simulink model "PI_current_IM"  (R2018b)
settings: Solver=ode45  StartTime=0.0  StopTime=2  RelTol=1e-7
values from neighbouring files (symbols this model uses):
  fs = 10000    [Motor_parameters_project.m]
  In = 189    [Motor_parameters_project.m]
  J = 0.0151    [Motor_parameters_project.m]
  Ki_d = 15.708    [Motor_parameters_project.m]
  Ki_q = 15.708    [Motor_parameters_project.m]
  Ki_speed = 2    [Motor_parameters_project.m]
  Kp_d = 2.5834    [Motor_parameters_project.m]
  Kp_q = 2.5834    [Motor_parameters_project.m]
  Kp_speed = 2    [Motor_parameters_project.m]
  landa_r = 0.0567    [Motor_parameters_project.m]
  Lm = 0.38e-3    (= 0.00038)    [Motor_parameters_project.m]
  Lr = Lm + Ldr    (= 0.00041116)    [Motor_parameters_project.m]
  Ls = Lm + Lds    (= 0.00041116)    [Motor_parameters_project.m]
  Omegae = 2*pi*fn    (= 364.424747816)    [Motor_parameters_project.m]
  p = 2.0    (= 2)    [Motor_parameters_project.m]
  Rr = 2.69e-3    (= 0.00269)    [Motor_parameters_project.m]
  Rs = 2.5e-3    (= 0.0025)    [Motor_parameters_project.m]
  T_rated = Pn/(2*pi*nn/60)    (= 30.0363631473)    [Motor_parameters_project.m]
  Ts = 1/fs    (= 0.0001)    [Motor_parameters_project.m]
  Udc = 36    [Motor_parameters_project.m]
  Un = 24/sqrt(3)    [Motor_parameters_project.m]
undefined symbols (not defined in the file or in its folder): sigbuilder_block
libraries: powerlib_meascontrol x1, powerlib x1
settings Model: Creator=estef  LastModifiedBy=estef

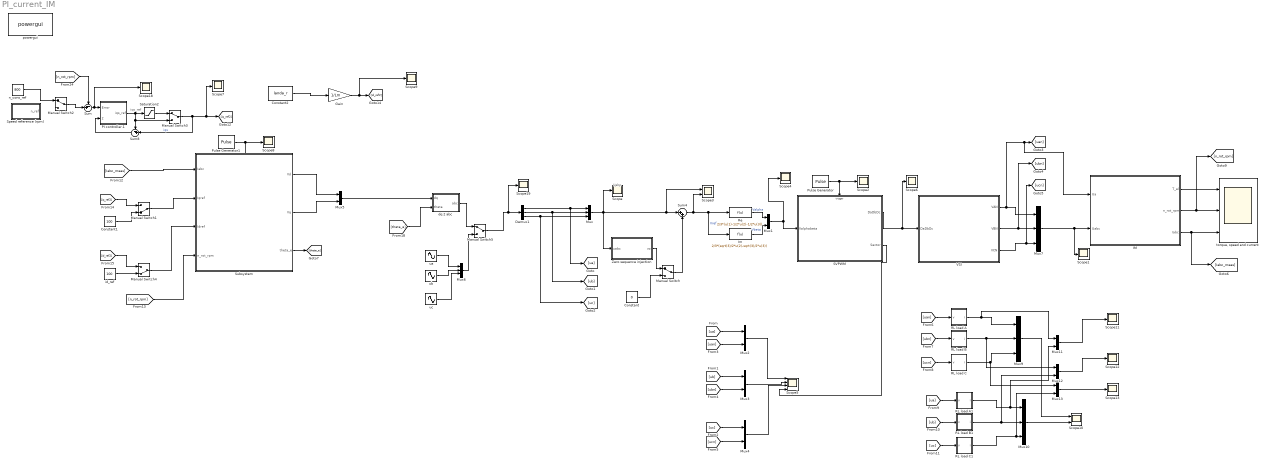
== system PI_current_IM ==
  note: Uabc
  note: iqs_ref
  Constant : Constant  Value=0
  Constant1 : Constant  Value=100
  Constant2 : Constant  Value=landa_r
  Demux1 : Demux  Outputs=3
  Gain : Gain  Gain=1/Lm
  "IM " : Subsystem
  Im : Fcn  Expr=2/3*(sqrt(3)/2*u(2)-sqrt(3)/2*u(3))
  Manual Switch{,2..3,5} (4 alike) : ManualSwitch
  Manual Switch1 : ManualSwitch  CurrentSetting=0
  Manual Switch4 : ManualSwitch  CurrentSetting=0
  Mux{,6..7,9..10} (5 alike) : Mux  Inputs=3
  Mux{1..5,11..13} (8 alike) : Mux  Inputs=2
  PI controller.1 : Subsystem
  Pulse Generator : DiscretePulseGenerator  PulseType=Time based  Period=1/fs  PulseWidth=50  PhaseDelay=1/fs/4
  Pulse Generator1 : DiscretePulseGenerator  PulseType=Time based  Period=2*Ts  PulseWidth=50  PhaseDelay=1/fs/4
  RL load A : Subsystem
  RL load A1 : Subsystem
  RL load B : Subsystem
  RL load B1 : Subsystem
  RL load C : Subsystem
  RL load C1 : Subsystem
  Re : Fcn  Expr=2/3*(u(1)-1/2*u(2)-1/2*u(3))
  "SVPWM " : Subsystem
  Saturation2 : Saturate  UpperLimit=In*sqrt(2)  LowerLimit=-In*sqrt(2)
  Scope{,1..2,4,6..9,11..13,18..19} (13 alike) : Scope
  Scope10 : Scope  NumInputPorts=2
  Scope3 : Scope  NumInputPorts=2
  Scope5 : Scope  NumInputPorts=4
  Speed reference (rpm) : Subsystem  Tag=STV Subsys  LoadFcn=sigbuilder_block('load');  StartFcn=sigbuilder_block('start');  StopFcn=sigbuilder_block('stop');  ClipboardFcn=sigbuilder_block('clipboard');  mask(Sigbuilder block){tuvar=[0:10]}
      mask help: Sigbuilder GUI
      mask init:
      | if ~strcmp(get_param(bdroot(gcbh),'SimulationStatus'),'stopped') tuvar = sigbuilder_block('maskInit'); end
      settings: CopyFcn=sigbuilder_block('copy');  DeleteFcn=sigbuilder_block('delete');  ModelCloseFcn=sigbuilder_block('modelClose');  PreSaveFcn=sigbuilder_block('preSave');  PauseFcn=sigbuilder_block('pause')  ContinueFcn=sigbuilder_block('continue')  NameChangeFcn=sigbuilder_block('namechange');  OpenFcn=sigbuilder_block('open',[176.25 175.5 550.5 399.75 ]);  CloseFcn=sigbuilder_block('close');
      mask Display: plot(0, 0, 100, 100,[2, 2, 32, 32, 2], [68, 8, 8, 68, 68],[32, 2], [38, 38], [32, 19, 2],[53, 60, 44], [32, 17, 17, 2],[16, 16, 31, 31]);txt = getActiveGroup(gcbh);text(2, 100, txt,'verticalAlignment', 'top');
  Subsystem : Subsystem
  Sum : Sum  Inputs=-+|
  Sum4 : Sum  Inputs=|++
  Sum8 : Sum  Inputs=-+|
  VSI : Subsystem
  Zero sequence injection : Subsystem
  dq 2 abc : Subsystem
  id_ref : Constant  Value=100
  n_cons_ref : Constant  Value=800
  powergui : powerlib/powergui  Priority=1  SimulationMode=Continuous  SampleTime=0.0000001  frequency=60  Iterations=50  frequencyindice=60  Pbase=100e6  ErrMax=1e-4  UnitsV=kV  UnitsW=MW  buscounter=0  FunctionMessages=off  echomessages=off  EnableUseOfTLC=off  CurrentSourceSwitches=off  DisableSnubberDevices=off  DisableRonSwitches=off  DisableVfSwitches=off  DisplayEquations=off  SolverType=Tustin/Backward Euler (TBE)  Interpol=off  ExternalGateDelay=off  methode=off  Ts=100  x0status=blocks  SPID=off  SwTol=0  HookPort=off  RestoreLinks=warning  ResistiveCurrentMeasurement=off  Frange=[0:2:500]  Ylog=off  Xlog=on  ShowGrid=off  save=off  variable=ZData  structure=0  ZoomFFT=off  StartTime=0.0  cycles=1  DisplayStyle=1  fundamental=60  FreqAxis=off  MaxFrequency=1000  frequencyindicesteady=1  RmsSteady=1  display=off
  "torque, speed and current " : Scope  NumInputPorts=3
  ua : Sin  Amplitude=sqrt(2)*Un  Frequency=Omegae  Phase=pi/2  SampleTime=0
  ub : Sin  Amplitude=sqrt(2)*Un  Frequency=Omegae  Phase=pi/2-120/180*pi  SampleTime=0
  uc : Sin  Amplitude=sqrt(2)*Un  Frequency=Omegae  Phase=pi/2-240/180*pi  SampleTime=0
  wires:
  Im/1 -> Mux1/2  "Vbeta"
  Re/1 -> Mux1/1  "Valpha"
  Sum4/1 -> Scope3/2, Im/1, Re/1  "Vref"
  Mux1/1 -> Scope4/1, "SVPWM "/1("Valphabeta ")
  Mux/1 -> Scope/1, Scope3/1, Sum4/1, Zero sequence injection/1(uabc)
  Manual Switch/1 -> Sum4/2
  Constant/1 -> Manual Switch/2
  Mux2/1 -> Scope5/1
  Mux3/1 -> Scope5/2
  Mux4/1 -> Scope5/3
  Zero sequence injection/1("vo ") -> Manual Switch/1
  [ua] -> Mux2/1
  [uan] -> Mux2/2
  [ubn] -> Mux3/2
  [ub] -> Mux3/1
  [ucn] -> Mux4/2
  [uc] -> Mux4/1
  RL load B/1(i) -> Mux12/1, Mux9/2
  RL load C/1(i) -> Mux13/1, Mux9/3
  RL load A/1(i) -> Mux11/1, Mux9/1
  [uan] -> RL load A/1(v)
  [ubn] -> RL load B/1(v)
  [ucn] -> RL load C/1(v)
  "SVPWM "/1(DaDbDc) -> Scope6/1, VSI/1(DaDbDc)
  Pulse Generator/1 -> Scope2/1, "SVPWM "/Trigger
  "SVPWM "/2("Sector ") -> Scope5/4
  [uc] -> RL load C1/1(v)
  [ub] -> RL load B1/1(v)
  [ua] -> RL load A1/1(v)
  RL load A1/1(i) -> Mux11/2, Mux10/1
  RL load C1/1(i) -> Mux13/2, Mux10/3
  RL load B1/1(i) -> Mux12/2, Mux10/2
  Mux9/1 -> Scope10/1
  Mux10/1 -> Scope10/2
  Mux11/1 -> Scope11/1
  Mux12/1 -> Scope12/1
  Mux13/1 -> Scope13/1
  "IM "/3(Iabc) -> [Iabc_meas], "torque, speed and current "/3
  "IM "/2("n_rot_rpm ") -> [n_rot_rpm], "torque, speed and current "/2
  "IM "/1(T_el) -> "torque, speed and current "/1
  VSI/1("VAN ") -> "IM "/1(Ua), [uan], Mux7/1
  VSI/2("VBN ") -> [ubn], Mux7/2
  VSI/3(VCN) -> [ucn], Mux7/3
  Mux7/1 -> Scope1/1, "IM "/2("Uabc ")
  Demux1/1 -> [ua], Mux/1
  Demux1/2 -> [ub], Mux/2
  Demux1/3 -> [uc], Mux/3
  Sum8/1 -> PI controller.1/2(anti-windup)
  Manual Switch3/1 -> Scope7/1, [iq_ref2], Sum8/2  "iqs"
  Saturation2/1 -> Manual Switch3/1
  [n_rot_rpm] -> Sum/1
  Sum/1 -> Scope18/1, PI controller.1/1(Error)
  PI controller.1/1(iqs_ref) -> Saturation2/1, Manual Switch3/2, Sum8/1
  Manual Switch2/1 -> Sum/2
  n_cons_ref/1 -> Manual Switch2/1
  Gain/1 -> Scope9/1, [id_ref2]
  Constant2/1 -> Gain/1
  Subsystem/1(Vd) -> Mux5/1
  Subsystem/2("Vq ") -> Mux5/2
  Mux5/1 -> dq 2 abc/1(dq)
  Subsystem/3("theta_e ") -> [theta_e]
  [Iabc_meas] -> Subsystem/1("Iabc ")
  id_ref/1 -> Manual Switch4/2
  [iq_ref2] -> Manual Switch1/1
  Constant1/1 -> Manual Switch1/2
  [id_ref2] -> Manual Switch4/1
  [n_rot_rpm] -> Subsystem/4("n_rot_rpm ")
  Pulse Generator1/1 -> Scope8/1
  [theta_e] -> dq 2 abc/2(theta)
  Manual Switch1/1 -> Subsystem/2("Iqref ")
  Manual Switch4/1 -> Subsystem/3("Idref ")
  ua/1 -> Mux6/1
  ub/1 -> Mux6/2
  uc/1 -> Mux6/3
  Mux6/1 -> Manual Switch5/2
  dq 2 abc/1(abc) -> Manual Switch5/1
  Manual Switch5/1 -> Scope19/1, Demux1/1

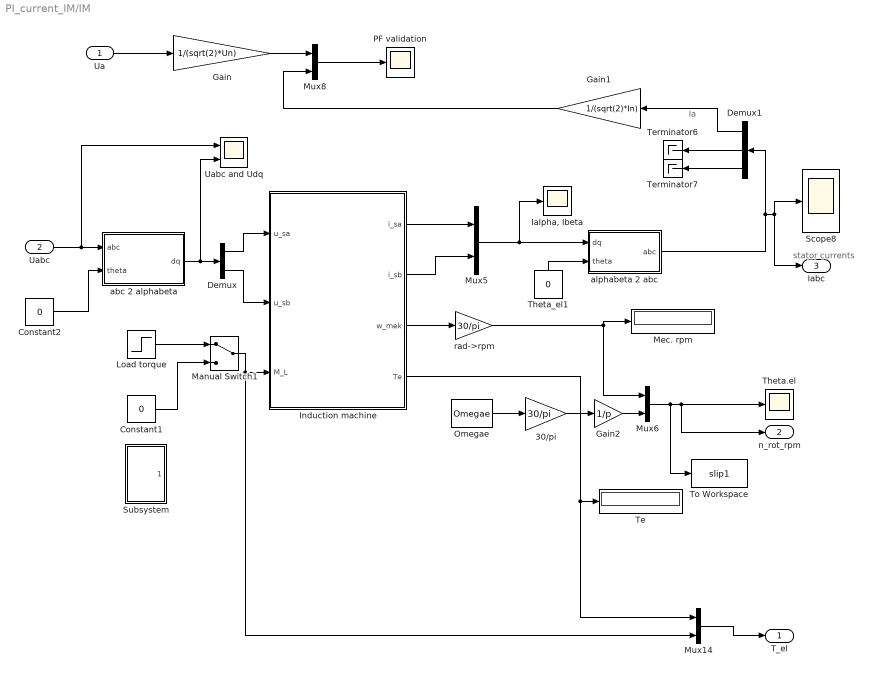
== system PI_current_IM/IM  ==
  note: stator currents
  note: Ia
  Ua : Inport
  "Uabc " : Inport  Port=2
  " PF validation" : Scope
  30/pi : Gain  Gain=30/pi
  Constant1 : Constant  Value=0
  Constant2 : Constant  Value=0
  Demux : Demux  Outputs=2
  Demux1 : Demux  Outputs=3
  Gain : Gain  Gain=1/(sqrt(2)*Un)
  Gain1 : Gain  Gain=1/(sqrt(2)*In)
  Gain2 : Gain  Gain=1/p
  "Ialpha, Ibeta" : Scope
  "Induction machine " : Subsystem
  Load torque : Step  Time=0.9  After=T_rated  SampleTime=0
  Manual Switch1 : ManualSwitch
  Mec. rpm : Display
  Mux{5..6,8,14} (4 alike) : Mux  Inputs=2
  Omegae : Constant  Value=Omegae
  Scope8 : Scope
  Subsystem : Subsystem
  Te : Display
  Terminator6 : Terminator
  Terminator7 : Terminator
  Theta.el : Scope
  Theta_el1 : Constant  Value=0
  To Workspace : ToWorkspace  VariableName=slip1  SaveFormat=Timeseries  SampleTime=-1
  Uabc and Udq : Scope  NumInputPorts=2
  abc 2 alphabeta : Subsystem
  alphabeta 2 abc : Subsystem
  rad->rpm : Gain  Gain=30/pi  SaturateOnIntegerOverflow=on  OutDataTypeStr=Inherit: Same as input  ParamDataTypeStr=Inherit: Same as input
  T_el : Outport
  "n_rot_rpm " : Outport  Port=2
  Iabc : Outport  Port=3
  wires:
  Demux1/2 -> Terminator6/1
  rad->rpm/1 -> Mec. rpm/1, Mux6/1
  "Induction machine "/4(Te) -> Mux14/1, Te/1
  Constant2/1 -> abc 2 alphabeta/2(theta)
  Mux8/1 -> " PF validation"/1
  Manual Switch1/1 -> Mux14/2, "Induction machine "/3(M_L)
  Gain/1 -> Mux8/1
  Mux6/1 -> To Workspace/1, "n_rot_rpm "/1, Theta.el/1
  alphabeta 2 abc/1(abc) -> Demux1/1, Iabc/1, Scope8/1
  abc 2 alphabeta/1(dq) -> Uabc and Udq/2, Demux/1
  Theta_el1/1 -> alphabeta 2 abc/2(theta)
  Mux14/1 -> T_el/1
  Mux5/1 -> "Ialpha, Ibeta"/1, alphabeta 2 abc/1(dq)
  "Induction machine "/1(i_sa) -> Mux5/1
  Gain1/1 -> Mux8/2
  Demux1/3 -> Terminator7/1
  30/pi/1 -> Gain2/1
  "Induction machine "/3(w_mek) -> rad->rpm/1
  "Induction machine "/2(i_sb) -> Mux5/2
  Demux1/1 -> Gain1/1
  Gain2/1 -> Mux6/2
  Demux/1 -> "Induction machine "/1(u_sa)
  Omegae/1 -> 30/pi/1
  Constant1/1 -> Manual Switch1/2
  Load torque/1 -> Manual Switch1/1
  Demux/2 -> "Induction machine "/2(u_sb)
  Ua/1 -> Gain/1
  "Uabc "/1 -> Uabc and Udq/1, abc 2 alphabeta/1(abc)

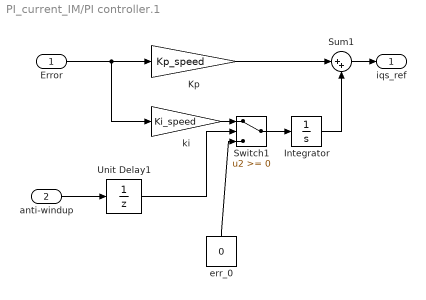
== system PI_current_IM/PI controller.1 ==
  Error : Inport
  anti-windup : Inport  Port=2
  Integrator : Integrator
  Kp : Gain  Gain=Kp_speed
  Sum1 : Sum  Inputs=|++
  Switch1 : Switch
  Unit Delay1 : UnitDelay  SampleTime=1/fs
  err_0 : Constant  Value=0
  ki : Gain  Gain=Ki_speed
  iqs_ref : Outport
  wires:
  Kp/1 -> Sum1/1
  Integrator/1 -> Sum1/2
  Sum1/1 -> iqs_ref/1
  Error/1 -> Kp/1, ki/1
  Unit Delay1/1 -> Switch1/2
  ki/1 -> Switch1/1
  Switch1/1 -> Integrator/1
  anti-windup/1 -> Unit Delay1/1
  err_0/1 -> Switch1/3

== system PI_current_IM/RL load A ==
  v : Inport
  1/L : Gain  Gain=1/Ls
  Integrator : Integrator
  R : Gain  Gain=Rs
  Sum : Sum  Inputs=|+-
  i : Outport
  wires:
  R/1 -> Sum/2
  Sum/1 -> 1/L/1
  1/L/1 -> Integrator/1
  Integrator/1 -> R/1, i/1
  v/1 -> Sum/1

== system PI_current_IM/RL load A1 ==
  v : Inport
  1/L : Gain  Gain=1/Ls
  Integrator : Integrator
  R : Gain  Gain=Rs
  Sum : Sum  Inputs=|+-
  i : Outport
  wires:
  v/1 -> Sum/1
  Integrator/1 -> i/1, R/1
  1/L/1 -> Integrator/1
  Sum/1 -> 1/L/1
  R/1 -> Sum/2

== system PI_current_IM/RL load B ==
  v : Inport
  1/L : Gain  Gain=1/Ls
  Integrator : Integrator
  R : Gain  Gain=Rs
  Sum : Sum  Inputs=|+-
  i : Outport
  wires:
  v/1 -> Sum/1
  Integrator/1 -> i/1, R/1
  1/L/1 -> Integrator/1
  Sum/1 -> 1/L/1
  R/1 -> Sum/2

== system PI_current_IM/RL load B1 ==
  v : Inport
  1/L : Gain  Gain=1/Ls
  Integrator : Integrator
  R : Gain  Gain=Rs
  Sum : Sum  Inputs=|+-
  i : Outport
  wires:
  R/1 -> Sum/2
  Sum/1 -> 1/L/1
  1/L/1 -> Integrator/1
  Integrator/1 -> R/1, i/1
  v/1 -> Sum/1

== system PI_current_IM/RL load C ==
  v : Inport
  1/L : Gain  Gain=1/Ls
  Integrator : Integrator
  R : Gain  Gain=Rs
  Sum : Sum  Inputs=|+-
  i : Outport
  wires:
  v/1 -> Sum/1
  Integrator/1 -> i/1, R/1
  1/L/1 -> Integrator/1
  Sum/1 -> 1/L/1
  R/1 -> Sum/2

== system PI_current_IM/RL load C1 ==
  v : Inport
  1/L : Gain  Gain=1/Ls
  Integrator : Integrator
  R : Gain  Gain=Rs
  Sum : Sum  Inputs=|+-
  i : Outport
  wires:
  R/1 -> Sum/2
  Sum/1 -> 1/L/1
  1/L/1 -> Integrator/1
  Integrator/1 -> R/1, i/1
  v/1 -> Sum/1

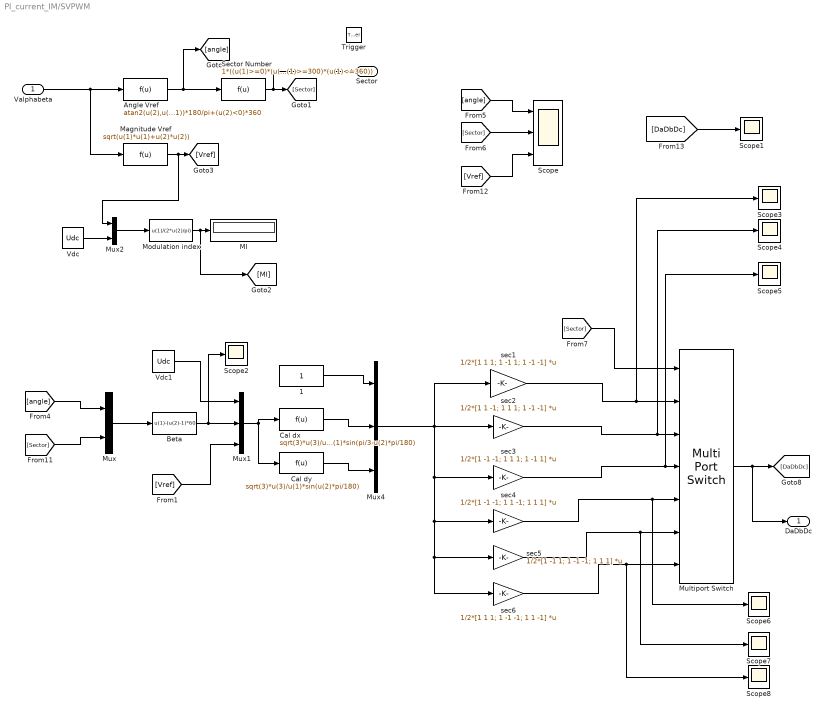
== system PI_current_IM/SVPWM  ==
  "Valphabeta " : Inport
  Trigger : TriggerPort  VariantControl=Variant  PortDimensions=1
  1 : Constant
  Angle Vref : Fcn  Expr=atan2(u(2),u(1))*180/pi+(u(2)<0)*360
  Beta : Fcn  Expr=u(1)-(u(2)-1)*60
  Cal dx : Fcn  Expr=sqrt(3)*u(3)/u(1)*sin(pi/3-u(2)*pi/180)
  Cal dy : Fcn  Expr=sqrt(3)*u(3)/u(1)*sin(u(2)*pi/180)
  MI : Display
  "Magnitude Vref " : Fcn  Expr=sqrt(u(1)*u(1)+u(2)*u(2))
  Modulation index : Fcn  Expr=u(1)/(2*u(2)/pi)
  Multiport Switch : MultiPortSwitch  Inputs=6
  Mux : Mux  Inputs=2
  Mux1 : Mux  Inputs=3
  Mux2 : Mux  Inputs=2
  Mux4 : Mux  Inputs=3
  Scope : Scope  NumInputPorts=3
  Scope{1..8} (8 alike) : Scope
  Sector Number : Fcn  Expr=1*((u(1)>=0)*(u(1)<60))+2*((u(1)>=60)*(u(1)<120))+3*((u(1)>=120)*(u(1)<180))+4*((u(1)>=180)*(u(1)<240))+5*((u(1)>=240)*(u(1)<300))+6*((u(1)>=300)*(u(1)<=360))
  Vdc : Constant  Value=Udc
  Vdc1 : Constant  Value=Udc
  sec1 : Gain  Gain=1/2*[1 1 1; 1 -1 1; 1 -1 -1]  Multiplication=Matrix(K*u)
  sec2 : Gain  Gain=1/2*[1 1 -1; 1 1 1; 1 -1 -1]  Multiplication=Matrix(K*u)
  sec3 : Gain  Gain=1/2*[1 -1 -1; 1 1 1; 1 -1 1]  Multiplication=Matrix(K*u)
  sec4 : Gain  Gain=1/2*[1 -1 -1; 1 1 -1; 1 1 1]  Multiplication=Matrix(K*u)
  sec5 : Gain  Gain=1/2*[1 -1 1; 1 -1 -1; 1 1 1]  Multiplication=Matrix(K*u)
  sec6 : Gain  Gain=1/2*[1 1 1; 1 -1 -1; 1 1 -1]  Multiplication=Matrix(K*u)
  DaDbDc : Outport
  "Sector " : Outport  Port=2
  wires:
  sec1/1 -> Scope3/1, Multiport Switch/2
  Modulation index/1 -> [MI], MI/1
  sec3/1 -> Scope5/1, Multiport Switch/4
  Mux2/1 -> Modulation index/1
  "Valphabeta "/1 -> "Magnitude Vref "/1, Angle Vref/1
  Sector Number/1 -> "Sector "/1, [Sector]
  sec4/1 -> Scope6/1, Multiport Switch/5
  "Magnitude Vref "/1 -> Mux2/1, [Vref]
  Angle Vref/1 -> [angle], Sector Number/1
  sec5/1 -> Scope7/1, Multiport Switch/6
  Vdc/1 -> Mux2/2
  sec2/1 -> Scope4/1, Multiport Switch/3
  sec6/1 -> Scope8/1, Multiport Switch/7
  [angle] -> Scope/1
  [Sector] -> Scope/2
  [Vref] -> Scope/3
  [DaDbDc] -> Scope1/1
  Mux/1 -> Beta/1
  [angle] -> Mux/1
  [Sector] -> Mux/2
  Beta/1 -> Scope2/1, Mux1/2
  Vdc1/1 -> Mux1/1
  [Vref] -> Mux1/3
  Mux1/1 -> Cal dx/1, Cal dy/1
  1/1 -> Mux4/1
  Cal dx/1 -> Mux4/2
  Cal dy/1 -> Mux4/3
  Mux4/1 -> sec6/1, sec5/1, sec4/1, sec3/1, sec2/1, sec1/1
  Multiport Switch/1 -> DaDbDc/1, [DaDbDc]
  [Sector] -> Multiport Switch/1

== system PI_current_IM/Speed reference (rpm) ==
  Demux : Demux  Tag=STV Demux  Outputs=1
  FromWs : FromWorkspace  Tag=STV FromWs  VariableName=tuvar  SampleTime=0
      SigBuilderData=|
      | common.afterFinalStr = 'Extrapolate'
      | common.sampleTime = 0
      | dataSet.timeRange = [0 10]
      | dataSet.name = 'Group 1'
      | sbobj.Groups.Name = 'Group 1'
      | sbobj.Groups.Signals.Name = 'n_ref'
      | sbobj.Groups.Signals.XData = [0 5 5.5 10]
      | sbobj.Groups.Signals.YData = [1000 998 500 500]
  n_ref : Outport  Tag=STV Outport
  wires:
  Demux/1 -> n_ref/1
  FromWs/1 -> Demux/1

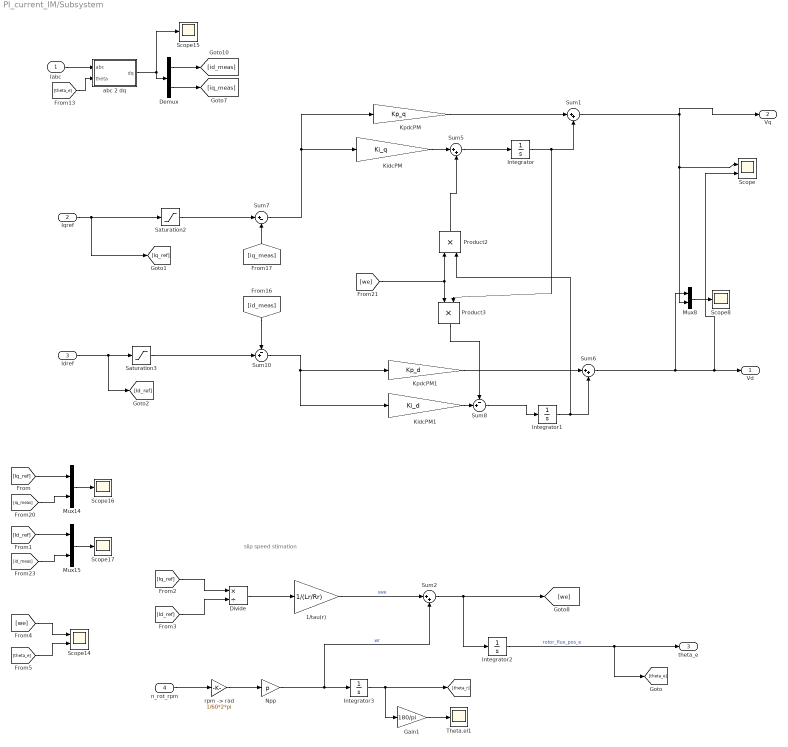
== system PI_current_IM/Subsystem ==
  note: slip speed stimation
  "Iabc " : Inport
  "Iqref " : Inport  Port=2
  "Idref " : Inport  Port=3
  "n_rot_rpm " : Inport  Port=4
  1/tau(r) : Gain  Gain=1/(Lr/Rr)
  Demux : Demux  Outputs=2
  Divide : Product  Inputs=*/
  Gain1 : Gain  Gain=180/pi
  Integrator{,1..3} (4 alike) : Integrator
  KidcPM : Gain  Gain=Ki_q
  KidcPM1 : Gain  Gain=Ki_d
  KpdcPM : Gain  Gain=Kp_q
  KpdcPM1 : Gain  Gain=Kp_d
  Mux14 : Mux  Inputs=2
  Mux15 : Mux  Inputs=2
  Mux8 : Mux  Inputs=2
  Npp : Gain  Gain=p  SaturateOnIntegerOverflow=on  OutDataTypeStr=Inherit: Same as input  ParamDataTypeStr=Inherit: Same as input
  Product2 : Product  SaturateOnIntegerOverflow=on  InputSameDT=on  OutDataTypeStr=Inherit: Same as first input
  Product3 : Product  SaturateOnIntegerOverflow=on  InputSameDT=on  OutDataTypeStr=Inherit: Same as first input
  Saturation2 : Saturate  UpperLimit=In*sqrt(2)  LowerLimit=-In*sqrt(2)
  Saturation3 : Saturate  UpperLimit=In*sqrt(2)  LowerLimit=-In*sqrt(2)
  Scope : Scope  NumInputPorts=2
  Scope14 : Scope  NumInputPorts=2
  Scope{8,15..17} (4 alike) : Scope
  Sum1 : Sum  Inputs=|++
  Sum10 : Sum  Inputs=-+|  SaturateOnIntegerOverflow=on  InputSameDT=on  OutDataTypeStr=Inherit: Same as first input
  Sum2 : Sum  Inputs=|++
  Sum5 : Sum  Inputs=|++  SaturateOnIntegerOverflow=on  InputSameDT=on  OutDataTypeStr=Inherit: Same as first input
  Sum6 : Sum  Inputs=|++
  Sum7 : Sum  Inputs=|+-  SaturateOnIntegerOverflow=on  InputSameDT=on  OutDataTypeStr=Inherit: Same as first input
  Sum8 : Sum  Inputs=-+|  SaturateOnIntegerOverflow=on  InputSameDT=on  OutDataTypeStr=Inherit: Same as first input
  Theta.el1 : Scope
  abc 2 dq : Subsystem
  "rpm -> rad" : Gain  Gain=1/60*2*pi  SaturateOnIntegerOverflow=on  OutDataTypeStr=Inherit: Same as input  ParamDataTypeStr=Inherit: Same as input
  Vd : Outport
  "Vq " : Outport  Port=2
  "theta_e " : Outport  Port=3
  wires:
  Mux8/1 -> Scope8/1
  Integrator2/1 -> [theta_e], "theta_e "/1  "rotor_flux_pos_e"
  Integrator1/1 -> Sum6/2, Product2/2
  KpdcPM1/1 -> Sum6/1
  [id_meas] -> Sum10/1
  Gain1/1 -> Theta.el1/1
  "n_rot_rpm "/1 -> "rpm -> rad"/1
  [we] -> Product2/1, Product3/1
  KpdcPM/1 -> Sum1/1
  Sum7/1 -> KidcPM/1, KpdcPM/1
  Divide/1 -> 1/tau(r)/1
  Integrator3/1 -> [theta_r], Gain1/1
  Npp/1 -> Integrator3/1, Sum2/2  "wr"
  1/tau(r)/1 -> Sum2/1  "swe"
  Integrator/1 -> Product3/2, Sum1/2
  Sum10/1 -> KidcPM1/1, KpdcPM1/1
  Sum8/1 -> Integrator1/1
  Sum2/1 -> Integrator2/1, [we]
  [iq_meas] -> Sum7/2
  "rpm -> rad"/1 -> Npp/1
  "Iqref "/1 -> [Iq_ref], Saturation2/1
  Sum5/1 -> Integrator/1
  Mux14/1 -> Scope16/1
  Mux15/1 -> Scope17/1
  "Idref "/1 -> [Id_ref], Saturation3/1
  [id_meas] -> Mux15/2
  [iq_meas] -> Mux14/2
  "Iabc "/1 -> abc 2 dq/1(abc)
  Demux/2 -> [iq_meas]
  [theta_e] -> abc 2 dq/2(theta)
  abc 2 dq/1(dq) -> Demux/1, Scope15/1
  Demux/1 -> [id_meas]
  Saturation2/1 -> Sum7/1
  Saturation3/1 -> Sum10/2
  [Iq_ref] -> Mux14/1
  [Id_ref] -> Mux15/1
  [Iq_ref] -> Divide/1
  [Id_ref] -> Divide/2
  [we] -> Scope14/1
  [theta_e] -> Scope14/2
  KidcPM/1 -> Sum5/1
  KidcPM1/1 -> Sum8/2
  Sum1/1 -> "Vq "/1, Mux8/2, Scope/1
  Sum6/1 -> Mux8/1, Scope/2, Vd/1
  Product3/1 -> Sum8/1
  Product2/1 -> Sum5/2

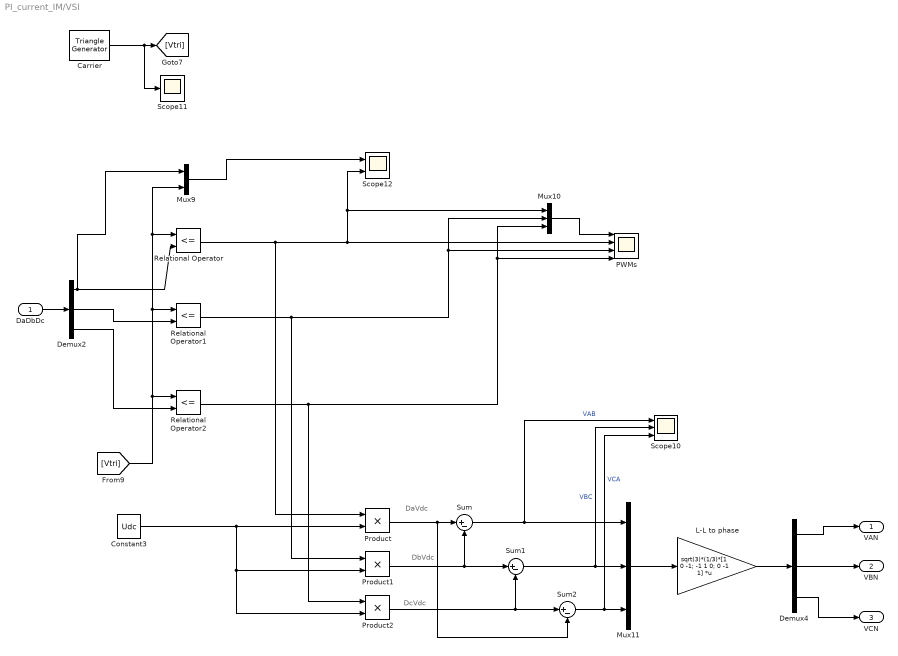
== system PI_current_IM/VSI ==
  note: DcVdc
  note: DaVdc
  note: DbVdc
  DaDbDc : Inport
  Carrier : powerlib_meascontrol/Pulse & Signal Generators/Triangle Generator  Freq=fs  Phase=0  Ts=0
      settings: SourceProductName=Simscape Electrical
  Constant3 : Constant  Value=Udc
  Demux2 : Demux  Outputs=3
  Demux4 : Demux  Outputs=3
  "L-L to phase " : Gain  Gain=sqrt(3)*(1/3)*[1 0 -1; -1 1 0; 0 -1 1]  Multiplication=Matrix(K*u)
  Mux10 : Mux  Inputs=3
  Mux11 : Mux  Inputs=3
  Mux9 : Mux  Inputs=2
  "PWMs " : Scope  NumInputPorts=4
  Product : Product
  Product1 : Product
  Product2 : Product
  Relational Operator : RelationalOperator  Operator=<=  OutDataTypeStr=boolean  RndMeth=Simplest
  Relational Operator1 : RelationalOperator  Operator=<=  OutDataTypeStr=boolean  RndMeth=Simplest
  Relational Operator2 : RelationalOperator  Operator=<=  OutDataTypeStr=boolean  RndMeth=Simplest
  Scope10 : Scope  NumInputPorts=3
  Scope11 : Scope
  Scope12 : Scope  NumInputPorts=2
  Sum : Sum  Inputs=|+-
  Sum1 : Sum  Inputs=|+-
  Sum2 : Sum  Inputs=|+-
  "VAN " : Outport
  "VBN " : Outport  Port=2
  VCN : Outport  Port=3
  wires:
  Sum1/1 -> Scope10/2, Mux11/2  "VBC"
  Carrier/1 -> Scope11/1, [Vtri]
  Mux10/1 -> "PWMs "/1
  Constant3/1 -> Product2/2, Product1/2, Product/2
  Demux4/3 -> VCN/1
  Demux2/2 -> Relational Operator1/2
  Demux4/2 -> "VBN "/1
  Product/1 -> Sum/1, Sum2/2
  [Vtri] -> Relational Operator1/1, Mux9/2, Relational Operator/1, Relational Operator2/1
  DaDbDc/1 -> Demux2/1
  Demux2/1 -> Mux9/1, Relational Operator/2
  Demux4/1 -> "VAN "/1
  Relational Operator/1 -> "PWMs "/2, Mux10/1, Scope12/2, Product/1
  Mux11/1 -> "L-L to phase "/1
  Product1/1 -> Sum1/1, Sum/2
  Product2/1 -> Sum2/1, Sum1/2
  Demux2/3 -> Relational Operator2/2
  Mux9/1 -> Scope12/1
  Relational Operator2/1 -> Product2/1, "PWMs "/4, Mux10/3
  Sum/1 -> Mux11/1, Scope10/1  "VAB"
  Sum2/1 -> Scope10/3, Mux11/3  "VCA"
  "L-L to phase "/1 -> Demux4/1
  Relational Operator1/1 -> "PWMs "/3, Mux10/2, Product1/1

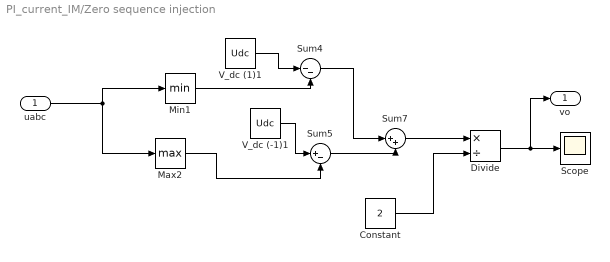
== system PI_current_IM/Zero sequence injection ==
  uabc : Inport
  Constant : Constant  Value=2
  Divide : Product  Inputs=*/
  Max2 : MinMax  Function=max
  Min1 : MinMax
  Scope : Scope
  Sum4 : Sum  Inputs=|--
  Sum5 : Sum  Inputs=|+-
  Sum7 : Sum  Inputs=|++
  V_dc (-1)1 : Constant  Value=Udc
  V_dc (1)1 : Constant  Value=Udc
  "vo " : Outport
  wires:
  Sum4/1 -> Sum7/1
  Sum7/1 -> Divide/1
  V_dc (-1)1/1 -> Sum5/1
  Min1/1 -> Sum4/2
  Constant/1 -> Divide/2
  Sum5/1 -> Sum7/2
  V_dc (1)1/1 -> Sum4/1
  Max2/1 -> Sum5/2
  uabc/1 -> Max2/1, Min1/1
  Divide/1 -> "vo "/1, Scope/1

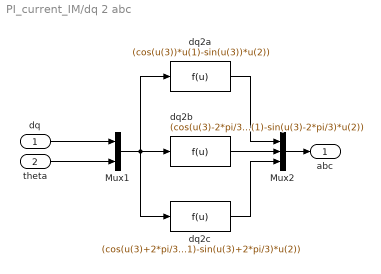
== system PI_current_IM/dq 2 abc ==
  dq : Inport
  theta : Inport  Port=2
  Mux1 : Mux  Inputs=2
  Mux2 : Mux  Inputs=3
  dq2a : Fcn  Expr=(cos(u(3))*u(1)-sin(u(3))*u(2))
  dq2b : Fcn  Expr=(cos(u(3)-2*pi/3)*u(1)-sin(u(3)-2*pi/3)*u(2))
  dq2c : Fcn  Expr=(cos(u(3)+2*pi/3)*u(1)-sin(u(3)+2*pi/3)*u(2))
  abc : Outport
  wires:
  Mux2/1 -> abc/1
  dq2b/1 -> Mux2/2
  dq2a/1 -> Mux2/1
  Mux1/1 -> dq2a/1, dq2c/1, dq2b/1
  theta/1 -> Mux1/2
  dq/1 -> Mux1/1
  dq2c/1 -> Mux2/3

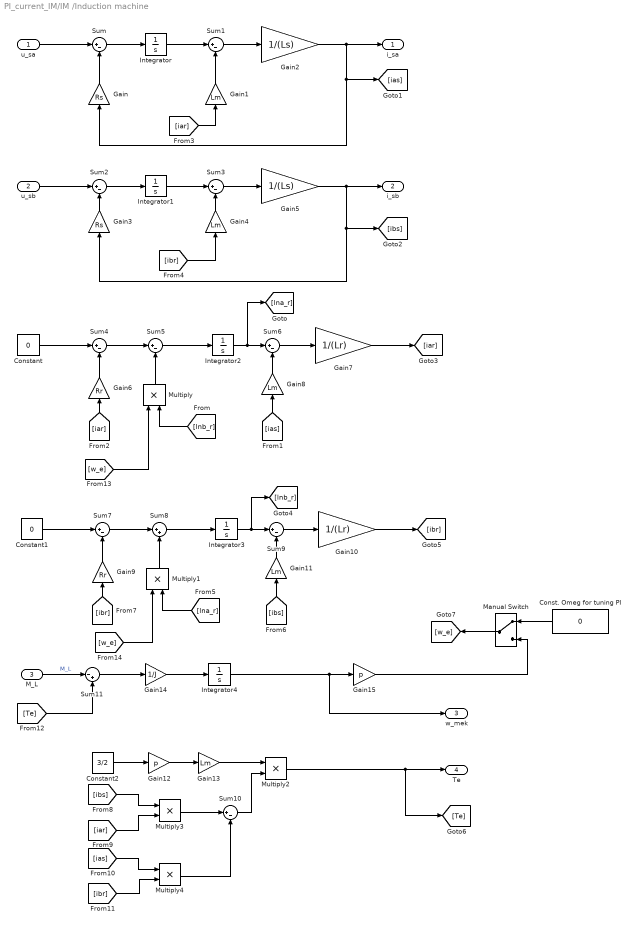
== system PI_current_IM/IM /Induction machine  ==
  u_sa : Inport
  u_sb : Inport  Port=2
  M_L : Inport  Port=3
  "Const. Omeg for tuning PI " : Constant  Value=0
  Constant : Constant  Value=0
  Constant1 : Constant  Value=0
  Constant2 : Constant  Value=3/2
  Gain : Gain  Gain=Rs
  Gain{1,4,8,11,13} (5 alike) : Gain  Gain=Lm
  Gain10 : Gain  Gain=1/(Lr)
  Gain12 : Gain  Gain=p
  Gain14 : Gain  Gain=1/J
  Gain15 : Gain  Gain=p
  Gain2 : Gain  Gain=1/(Ls)
  Gain3 : Gain  Gain=Rs
  Gain5 : Gain  Gain=1/(Ls)
  Gain6 : Gain  Gain=Rr
  Gain7 : Gain  Gain=1/(Lr)
  Gain9 : Gain  Gain=Rr
  Integrator{,1..4} (5 alike) : Integrator
  Manual Switch : ManualSwitch
  Multiply{,1..4} (5 alike) : Product
  Sum{,1..7,9..10} (10 alike) : Sum  Inputs=|+-
  Sum11 : Sum  Inputs=|-+
  Sum8 : Sum  Inputs=|++
  i_sa : Outport
  i_sb : Outport  Port=2
  w_mek : Outport  Port=3
  Te : Outport  Port=4
  wires:
  u_sa/1 -> Sum/1
  Gain/1 -> Sum/2
  Sum/1 -> Integrator/1
  Integrator/1 -> Sum1/1
  Gain1/1 -> Sum1/2
  Sum1/1 -> Gain2/1
  Gain2/1 -> [ias], Gain/1, i_sa/1
  Gain3/1 -> Sum2/2
  u_sb/1 -> Sum2/1
  Sum3/1 -> Gain5/1
  Gain4/1 -> Sum3/2
  Gain5/1 -> i_sb/1, [ibs], Gain3/1
  Sum2/1 -> Integrator1/1
  Integrator1/1 -> Sum3/1
  Constant/1 -> Sum4/1
  Gain6/1 -> Sum4/2
  Sum4/1 -> Sum5/1
  [lnb_r] -> Multiply/2
  Sum5/1 -> Integrator2/1
  Gain8/1 -> Sum6/2
  [ias] -> Gain8/1
  Integrator2/1 -> [lna_r], Sum6/1
  Sum6/1 -> Gain7/1
  Multiply/1 -> Sum5/2
  Gain7/1 -> [iar]
  [iar] -> Gain6/1
  [ibr] -> Gain4/1
  [iar] -> Gain1/1
  Gain11/1 -> Sum9/2
  Gain10/1 -> [ibr]
  [ibr] -> Gain9/1
  [ibs] -> Gain11/1
  Multiply1/1 -> Sum8/2
  Integrator3/1 -> [lnb_r], Sum9/1
  Sum7/1 -> Sum8/1
  [lna_r] -> Multiply1/2
  Gain9/1 -> Sum7/2
  Sum9/1 -> Gain10/1
  Sum8/1 -> Integrator3/1
  Constant1/1 -> Sum7/1
  Gain13/1 -> Multiply2/1
  Sum10/1 -> Multiply2/2
  [ibs] -> Multiply3/1
  [iar] -> Multiply3/2
  Multiply3/1 -> Sum10/1
  [ias] -> Multiply4/1
  [ibr] -> Multiply4/2
  Multiply4/1 -> Sum10/2
  Constant2/1 -> Gain12/1
  Gain12/1 -> Gain13/1
  Multiply2/1 -> [Te], Te/1
  [Te] -> Sum11/2
  M_L/1 -> Sum11/1  "M_L"
  Sum11/1 -> Gain14/1
  Gain14/1 -> Integrator4/1
  [w_e] -> Multiply/1
  [w_e] -> Multiply1/1
  "Const. Omeg for tuning PI "/1 -> Manual Switch/1
  Gain15/1 -> Manual Switch/2
  Manual Switch/1 -> [w_e]
  Integrator4/1 -> w_mek/1, Gain15/1

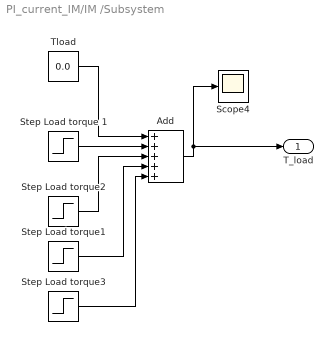
== system PI_current_IM/IM /Subsystem ==
  Add : Sum  Inputs=+++++
  Scope4 : Scope
  Step Load torque 1 : Step  Time=0.9  After=5  SampleTime=0
  Step Load torque1 : Step  Time=1.5  After=8  SampleTime=0
  Step Load torque2 : Step  Time=1.2  After=8  SampleTime=0
  Step Load torque3 : Step  Time=1.8  After=10  SampleTime=0
  Tload : Constant  Value=0.0
  T_load : Outport
  wires:
  Add/1 -> T_load/1, Scope4/1
  Step Load torque 1/1 -> Add/2
  Tload/1 -> Add/1
  Step Load torque2/1 -> Add/3
  Step Load torque1/1 -> Add/4
  Step Load torque3/1 -> Add/5

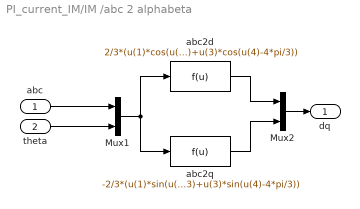
== system PI_current_IM/IM /abc 2 alphabeta ==
  abc : Inport
  theta : Inport  Port=2
  Mux1 : Mux  Inputs=2
  Mux2 : Mux  Inputs=2
  abc2d : Fcn  Expr=2/3*(u(1)*cos(u(4))+u(2)*cos(u(4)-2*pi/3)+u(3)*cos(u(4)-4*pi/3))
  abc2q : Fcn  Expr=-2/3*(u(1)*sin(u(4))+u(2)*sin(u(4)-2*pi/3)+u(3)*sin(u(4)-4*pi/3))
  dq : Outport
  wires:
  abc/1 -> Mux1/1
  theta/1 -> Mux1/2
  Mux1/1 -> abc2d/1, abc2q/1
  abc2d/1 -> Mux2/1
  abc2q/1 -> Mux2/2
  Mux2/1 -> dq/1

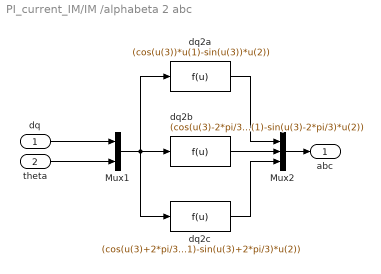
== system PI_current_IM/IM /alphabeta 2 abc ==
  dq : Inport
  theta : Inport  Port=2
  Mux1 : Mux  Inputs=2
  Mux2 : Mux  Inputs=3
  dq2a : Fcn  Expr=(cos(u(3))*u(1)-sin(u(3))*u(2))
  dq2b : Fcn  Expr=(cos(u(3)-2*pi/3)*u(1)-sin(u(3)-2*pi/3)*u(2))
  dq2c : Fcn  Expr=(cos(u(3)+2*pi/3)*u(1)-sin(u(3)+2*pi/3)*u(2))
  abc : Outport
  wires:
  Mux2/1 -> abc/1
  dq2b/1 -> Mux2/2
  dq2a/1 -> Mux2/1
  Mux1/1 -> dq2a/1, dq2c/1, dq2b/1
  theta/1 -> Mux1/2
  dq/1 -> Mux1/1
  dq2c/1 -> Mux2/3

== system PI_current_IM/Subsystem/abc 2 dq ==
  abc : Inport
  theta : Inport  Port=2
  Mux1 : Mux  Inputs=2
  Mux2 : Mux  Inputs=2
  abc2d : Fcn  Expr=2/3*(u(1)*cos(u(4))+u(2)*cos(u(4)-2*pi/3)+u(3)*cos(u(4)-4*pi/3))
  abc2q : Fcn  Expr=-2/3*(u(1)*sin(u(4))+u(2)*sin(u(4)-2*pi/3)+u(3)*sin(u(4)-4*pi/3))
  dq : Outport
  wires:
  abc/1 -> Mux1/1
  theta/1 -> Mux1/2
  Mux1/1 -> abc2d/1, abc2q/1
  abc2d/1 -> Mux2/1
  abc2q/1 -> Mux2/2
  Mux2/1 -> dq/1
